simulink model "TST00_LeggeDecadimentoRadioattivo"  (R2023a)
settings: Solver=VariableStepAuto  StartTime=0.0  StopTime=5370  RelTol=1e-3
settings Model: Creator=admin  LastModifiedBy=admin

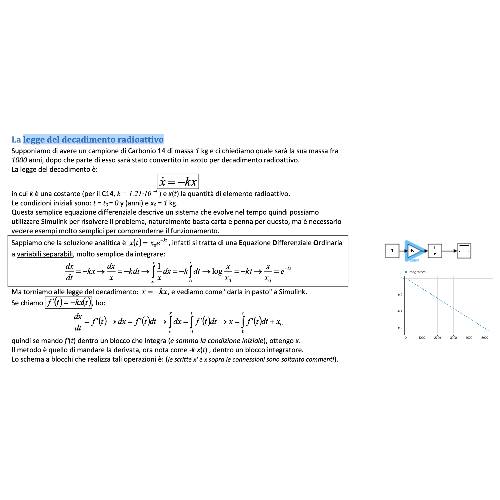
[thumbnail: Simulink's stored preview of the top-level diagram]
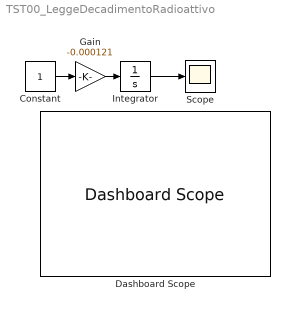
== system TST00_LeggeDecadimentoRadioattivo ==
  Constant : Constant
  Dashboard Scope : DashboardScope
  Gain : Gain  Gain=-0.000121
  Integrator : Integrator
  Scope : Scope
  wires:
  Integrator/1 -> Scope/1
  Constant/1 -> Gain/1
  Gain/1 -> Integrator/1
